simulink model "control_and_guidance"  (Simulink 7.6)
settings: Solver=FixedStepDiscrete  StartTime=0.0  StopTime=Tfin  FixedStep=Ts  RelTol=1e-3
settings Model: Creator=borjafons  LastModifiedBy=frafonal
settings OptimizationCC: InlineParams=on  OptimizeModelRefInitCode=on  LifeSpan=1
settings DebuggingCC: FcnCallInpInsideContextMsg=Enable All
settings RTWCC: SystemTargetFile=ert.tlc  GenCodeOnly=on  TemplateMakefile=ert_default_tmf  Description=Embedded Coder  ProcessScript=ert_make_rtw_hook
settings CodeAppCC: IgnoreCustomStorageClasses=off
settings ERTTargetCC: MultiwordLength=2048  GenerateSampleERTMain=on  SupportAbsoluteTime=off  SupportComplex=off  InlinedParameterPlacement=NonHierarchical  ERTCustomFileTemplate=example_file_process.tlc  ConvertIfToSwitch=off

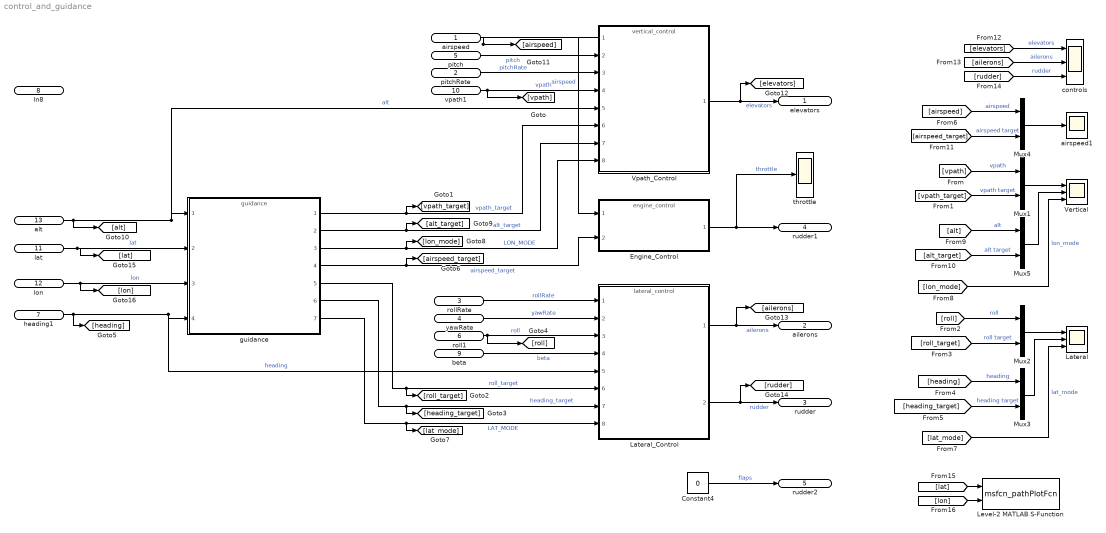
== system control_and_guidance ==
  airspeed : Inport
  pitchRate : Inport  Port=2
  rollRate : Inport  Port=3
  yawRate : Inport  Port=4
  pitch : Inport  Port=5
  roll1 : Inport  Port=6
  heading1 : Inport  Port=7
  In8 : Inport  Port=8
  beta : Inport  Port=9
  vpath1 : Inport  Port=10
  lat : Inport  Port=11
  lon : Inport  Port=12
  alt : Inport  Port=13
  Constant4 : Constant  Value=0  OutDataTypeStr=double
  Engine_Control : ModelReference  ModelNameDialog=engine_control  SimulationMode=Normal  ModelReferenceVersion=1.98  CopyOfModelName=engine_control  DefaultDataLogging=on
  Lateral : Scope  NumInputPorts=3
      settings: YMin=-9~178~0  YMax=4~185.5~1  SaveName=ScopeData2  SampleInput=on  SampleTime=Ts
  Lateral_Control : ModelReference  ModelNameDialog=lateral_control  SimulationMode=Normal  ModelReferenceVersion=1.92  CopyOfModelName=lateral_control  DefaultDataLogging=on
  Level-2 MATLAB S-Function : M-S-Function  FunctionName=msfcn_pathPlotFcn  Parameters=wp
      mask Display:
      | disp('plot path')
      | port_label('input', 1, 'lat')
      | port_label('input', 2, 'lon')
  Mux{1..5} (5 alike) : Mux  Inputs=2
  Vertical : Scope  NumInputPorts=3
      settings: YMin=-0.1~1994~-1  YMax=0.9~2000~1  SampleInput=on  SampleTime=Ts
  Vpath_Control : ModelReference  ModelNameDialog=vertical_control  SimulationMode=Normal  ModelReferenceVersion=1.100  CopyOfModelName=vertical_control  DefaultDataLogging=on
  airspeed1 : Scope
      settings: YMin=110  YMax=113  SaveName=ScopeData4  SampleInput=on  SampleTime=Ts
  controls : Scope  NumInputPorts=3
      settings: YMin=-0.007~-0.03~-0.2  YMax=-0.001~0.03~0.2  SaveName=ScopeData3  SampleInput=on  SampleTime=Ts
  guidance : ModelReference  ModelNameDialog=guidance  SimulationMode=Normal  ModelReferenceVersion=1.136  CopyOfModelName=guidance  DefaultDataLogging=on
  throttle : Scope
      settings: YMin=0.2  YMax=0.9  SampleInput=on  SampleTime=Ts
  elevators : Outport
  ailerons : Outport  Port=2
  rudder : Outport  Port=3
  rudder1 : Outport  Port=4
  rudder2 : Outport  Port=5
  wires:
  airspeed/1 -> Vpath_Control/1, Engine_Control/1, [airspeed]  "airspeed"
  pitch/1 -> Vpath_Control/2  "pitch"
  pitchRate/1 -> Vpath_Control/3  "pitchRate"
  vpath1/1 -> [vpath], Vpath_Control/4  "vpath"
  rollRate/1 -> Lateral_Control/1  "rollRate"
  yawRate/1 -> Lateral_Control/2  "yawRate"
  Vpath_Control/1 -> elevators/1, [elevators]  "elevators"
  Lateral_Control/1 -> ailerons/1, [ailerons]  "ailerons"
  Lateral_Control/2 -> rudder/1, [rudder]  "rudder"
  heading1/1 -> [heading], Lateral_Control/5, guidance/4  "heading"
  beta/1 -> Lateral_Control/4  "beta"
  roll1/1 -> Lateral_Control/3, [roll]  "roll"
  Mux1/1 -> Vertical/1
  [vpath_target] -> Mux1/2  "vpath target"
  [vpath] -> Mux1/1  "vpath"
  [roll_target] -> Mux2/2  "roll target"
  [roll] -> Mux2/1  "roll"
  Mux3/1 -> Lateral/2
  [heading_target] -> Mux3/2  "heading target"
  [heading] -> Mux3/1  "heading"
  [elevators] -> controls/1  "elevators"
  [ailerons] -> controls/2  "ailerons"
  [rudder] -> controls/3  "rudder"
  alt/1 -> [alt], guidance/1, Vpath_Control/5  "alt"
  [lon_mode] -> Vertical/3  "lon_mode"
  Mux5/1 -> Vertical/2
  [alt_target] -> Mux5/2  "alt target"
  [alt] -> Mux5/1  "alt"
  Mux2/1 -> Lateral/1
  [lat_mode] -> Lateral/3  "lat_mode"
  Engine_Control/1 -> rudder1/1, throttle/1  "throttle"
  Constant4/1 -> rudder2/1  "flaps"
  Mux4/1 -> airspeed1/1
  [airspeed_target] -> Mux4/2  "airspeed target"
  [airspeed] -> Mux4/1  "airspeed"
  lat/1 -> [lat], guidance/2  "lat"
  lon/1 -> guidance/3, [lon]  "lon"
  guidance/1 -> Vpath_Control/6, [vpath_target]  "vpath_target"
  guidance/2 -> Vpath_Control/7, [alt_target]  "alt_target"
  guidance/3 -> Vpath_Control/8, [lon_mode]  "LON_MODE"
  guidance/4 -> Engine_Control/2, [airspeed_target]  "airspeed_target"
  guidance/5 -> Lateral_Control/6, [roll_target]  "roll_target"
  guidance/6 -> Lateral_Control/7, [heading_target]  "heading_target"
  guidance/7 -> Lateral_Control/8, [lat_mode]  "LAT_MODE"
  [lat] -> Level-2 MATLAB S-Function/1
  [lon] -> Level-2 MATLAB S-Function/2
